simulink model "Part1_I"  (R2023b)
settings: Solver=VariableStepAuto  StartTime=0.0  StopTime=1  RelTol=1e-3
undefined symbols (not defined in the file): null
libraries: commchan3 x1, dspfdesign x1
settings Model: Creator=henry  LastModifiedBy=henry

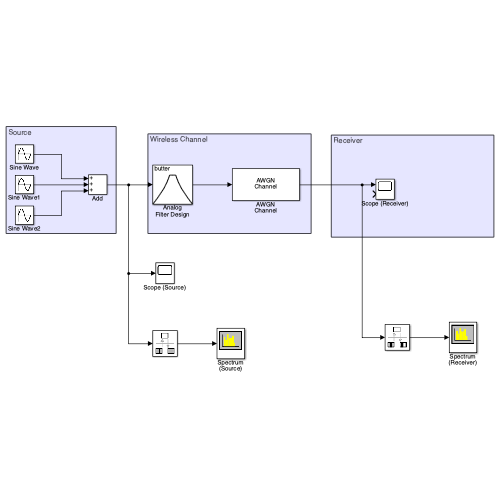
[thumbnail: Simulink's stored preview of the top-level diagram]
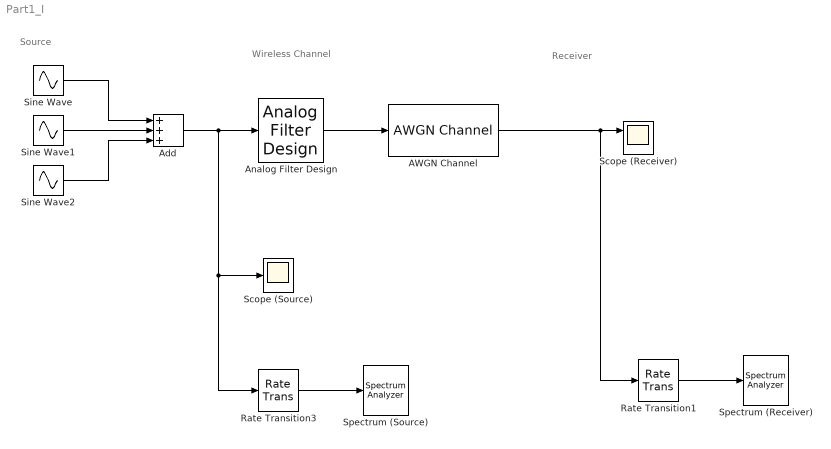
== system Part1_I ==
  note: Receiver
  note: Wireless Channel
  note: Source
  AWGN Channel : commchan3/AWGN Channel  LegacyMode=off  NoiseMethod=Variance  noiseMode="Signal to noise ratio  (SNR)"  EbNo=10  EsNo=10  SNR=10  BitsPerSymbol=1  SignalPower=1  SamplesPerSymbol=1  SymbolPeriod=1  VarianceSource=Parameter  Variance=1e-3  RandomStream=mt19937ar with seed  Seed=100  SimulateUsing=Interpreted execution
  Add : Sum  Inputs=+++
  Analog Filter Design : dspfdesign/Analog Filter Design  method=Butterworth  filttype=Bandpass  N=8  Wlo=2e4*pi  Whi=4e4*pi  Rp=2  Rs=40
  Rate Transition1 : RateTransition  OutPortSampleTime=1/50000
  Rate Transition3 : RateTransition  OutPortSampleTime=1/50000
  Scope (Receiver) : Scope  NumInputPorts=2
  Scope (Source) : Scope
  Sine Wave : Sin  Amplitude=0.5  Frequency=1000*pi  SampleTime=0
  Sine Wave1 : Sin  Amplitude=0.2  Frequency=600*pi  SampleTime=0
  Sine Wave2 : Sin  Amplitude=0.3  Frequency=1200*pi  SampleTime=0
  Spectrum (Receiver) : SpectrumAnalyzer  WindowPosition=[260.000000,200.000000,800.000000,500.000000,]  ScopeFrameLocation=window  YLimits=[null,null]
  Spectrum (Source) : SpectrumAnalyzer  WindowPosition=[320.000000,200.000000,800.000000,500.000000,]  ScopeFrameLocation=window  YLimits=[-40.72099746,17.78992482]
  wires:
  Sine Wave1/1 -> Add/2
  Sine Wave/1 -> Add/1
  Sine Wave2/1 -> Add/3
  Analog Filter Design/1 -> AWGN Channel/1
  Rate Transition3/1 -> Spectrum (Source)/1
  Rate Transition1/1 -> Spectrum (Receiver)/1
  AWGN Channel/1 -> Rate Transition1/1, Scope (Receiver)/1
  Add/1 -> Scope (Source)/1, Rate Transition3/1, Analog Filter Design/1
